simulink model "TX_PM_MODEL"  (R2024a)
settings: Solver=VariableStepAuto  StartTime=0.0  StopTime=1e-3  FixedStep=1e-9  RelTol=1e-3
values from neighbouring files (symbols this model uses):
  Cs = 12.5e-12    (= 1.25e-11)    [Oscillator_Setup.m]
  deltaVOSC = 0.5    [Oscillator_Setup.m]
  I0 = 100e-6    (= 0.0001)    [Oscillator_Setup.m]
  R = 0.2    [TX_PM_MODEL_Setup.m]
  Rf = 1e9    (= 1000000000)    [Oscillator_Setup.m]
  VDD = 5    [Oscillator_Setup.m]    (also in TX_PM_MODEL_Setup.m = 10)
  Vh = VDD - deltaVOSC    (= 4.5)    [Oscillator_Setup.m]
  Vl = deltaVOSC    (= 0.5)    [Oscillator_Setup.m]
undefined symbols (not defined in the file or in its folder): VDD_DRIVE
libraries: fl_lib x12, nesl_utility x7, ee_lib x1, dspsigops x1, spsTriangleGeneratorLib x1
settings Model: Creator=cian.odonnell  LastModifiedBy=cian.odonnell
settings SolverCC: EnableFixedStepZeroCrossing=on

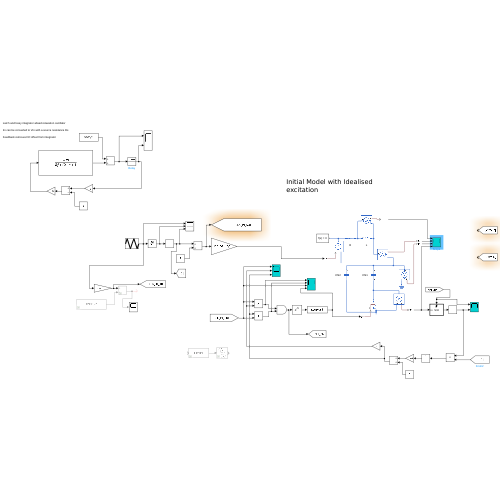
[thumbnail: Simulink's stored preview of the top-level diagram]
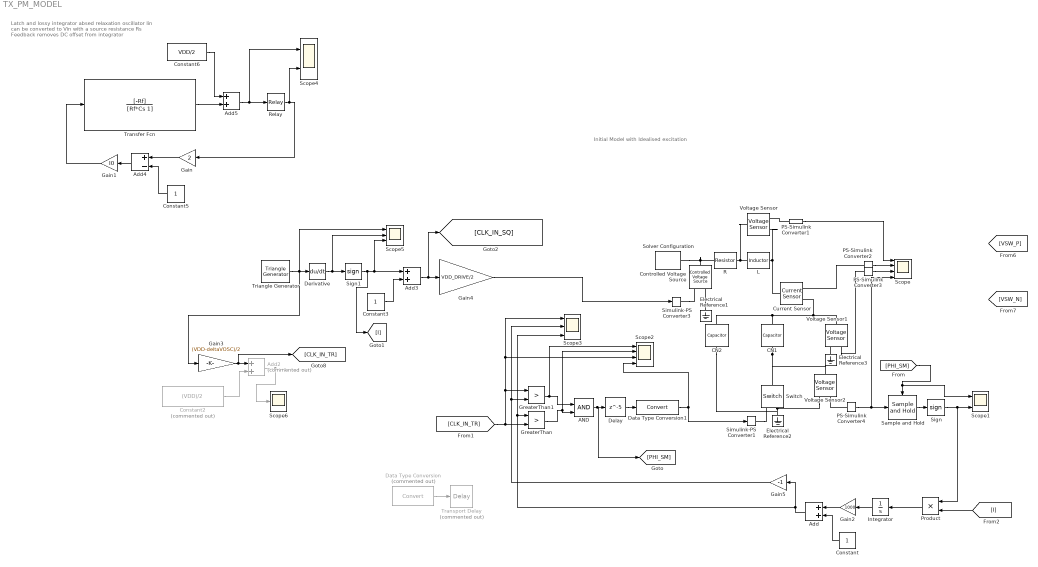
== system TX_PM_MODEL ==
  note: Initial Model with Idealised excitation
  note: Latch and lossy integrator absed relaxation oscillator
      |
      | Iin can be converted to Vin with a source resistance Rs
      |
      | Feedback removes DC offset from integrator
  AND : Logic  IconShape=distinctive  AllPortsSameDT=off  OutDataTypeStr=boolean
  Add : Sum
  Add2 : Sum  Commented=on
  Add3 : Sum
  Add4 : Sum  Inputs=+-
  Add5 : Sum
  CN1 : fl_lib/Electrical/Electrical Elements/Capacitor  c=3e-9 F  r=1e-6 Ohm  g=0 1/Ohm  i_specify=off  i_priority=None  i=0 A  i_nominal_specify=off  i_nominal_value=1  i_nominal_unit=A  v_specify=off  v_priority=None  v=0 V  v_nominal_specify=off  v_nominal_value=1  v_nominal_unit=V  vc_specify=off  vc_priority=High  vc=0 V  vc_nominal_specify=off  vc_nominal_value=1  vc_nominal_unit=V
  CN2 : fl_lib/Electrical/Electrical Elements/Capacitor  c=3e-9 F  r=1e-6 Ohm  g=0 1/Ohm  i_specify=off  i_priority=None  i=0 A  i_nominal_specify=off  i_nominal_value=1  i_nominal_unit=A  v_specify=off  v_priority=None  v=0 V  v_nominal_specify=off  v_nominal_value=1  v_nominal_unit=V  vc_specify=off  vc_priority=High  vc=0 V  vc_nominal_specify=off  vc_nominal_value=1  vc_nominal_unit=V
  Constant : Constant
  Constant2 : Constant  Commented=on  Value=(VDD)/2
  Constant3 : Constant
  Constant5 : Constant
  Constant6 : Constant  Value=VDD/2
  Controlled Voltage Source : fl_lib/Electrical/Electrical Sources/Controlled Voltage Source
  Current Sensor : fl_lib/Electrical/Electrical Sensors/Current Sensor
  Data Type Conversion : DataTypeConversion  Commented=on  SaturateOnIntegerOverflow=off  RndMeth=Floor
  Data Type Conversion1 : DataTypeConversion  SaturateOnIntegerOverflow=off  RndMeth=Floor
  Delay : Delay  DelayLength=5  SampleTime=1e-9
  Derivative : Derivative
  Electrical Reference1 : fl_lib/Electrical/Electrical Elements/Electrical Reference
  Electrical Reference2 : fl_lib/Electrical/Electrical Elements/Electrical Reference
  Electrical Reference3 : fl_lib/Electrical/Electrical Elements/Electrical Reference
  Gain : Gain  Gain=2
  Gain1 : Gain  Gain=I0
  Gain2 : Gain  Gain=1000
  Gain3 : Gain  Gain=(VDD-deltaVOSC)/2
  Gain4 : Gain  Gain=VDD_DRIVE/2
  Gain5 : Gain  Gain=-1
  GreaterThan : RelationalOperator  Operator=>  OutDataTypeStr=boolean  RndMeth=Simplest  InputSameDT=off
  GreaterThan1 : RelationalOperator  Operator=>  OutDataTypeStr=boolean  RndMeth=Simplest  InputSameDT=off
  Integrator : Integrator
  L : ee_lib/Passive/Inductor  l=L H  enable_L_tol=ee.enum.toleranceApplication.none  L_tol=20  tol_distribution=ee.enum.toleranceDistribution.uniform  nSigma=4  r=0 Ohm  g=1e-9 1/Ohm  enable_operating_limits=ee.enum.enable.no  operating_limit_action=ee.enum.passive.reportOpLim.warn  max_working_current=1 A  power_rating=1 W  enable_faults=ee.enum.enable.no  fault_action=simscape.enum.assert.action.none  lambdaPercent=50  k_faulted=0.9999  turnsShort=ee.enum.passive.inductor.turnsShortOption.no  openCct=ee.enum.enable.no  groundShort=ee.enum.passive.inductor.groundShortOption.no  groundShortG=0 1/Ohm  tau_fault=1e-3 s  fault_trigger=ee.enum.faults.faultTrigger.temporal  t_fault=1 s  max_permissible_voltage=100 V  n_fail_on_voltage=1  max_permissible_current=1 A  t_fail_on_current=1 s  i_L_specify=off  i_L_priority=High  i_L=0 A  i_L_nominal_specify=off  i_L_nominal_value=1  i_L_nominal_unit=A  faulted_specify=off  faulted_priority=None  faulted=0
  PS-Simulink Converter{1..4} (4 alike) : nesl_utility/PS-Simulink Converter  PhysicalDomain=network_engine_domain  SubClassName=ps_output  LeftPortType=input  RightPortType=output  PseudoPeriodic=off  Frequencies=[]  VectorFormat=inherit  Unit=inherit  AffineConversion=off
  Product : Product
  R : fl_lib/Electrical/Electrical Elements/Resistor  R=R Ohm  i_specify=off  i_priority=None  i=0 A  i_nominal_specify=off  i_nominal_value=1  i_nominal_unit=A  v_specify=off  v_priority=None  v=0 V  v_nominal_specify=off  v_nominal_value=1  v_nominal_unit=V
  Relay : Relay  OnSwitchValue=Vh  OffSwitchValue=Vl
  Sample and Hold : dspsigops/Sample and Hold  trig=Rising edge  initCond=0  latchinput=off
  Scope : Scope  NumInputPorts=4
  Scope1 : Scope  NumInputPorts=2
  Scope2 : Scope  NumInputPorts=4
  Scope3 : Scope  NumInputPorts=3
  Scope4 : Scope  NumInputPorts=2
  Scope5 : Scope  NumInputPorts=3
  Scope6 : Scope
  Sign : Signum
  Sign1 : Signum
  Simulink-PS Converter1 : nesl_utility/Simulink-PS Converter  PhysicalDomain=network_engine_domain  SubClassName=ps_input  LeftPortType=input  RightPortType=output  PseudoPeriodic=off  Frequencies=[]  NoiseDistribution=none  NoiseParameters=[]  Unit=1  AffineConversion=off  FilteringAndDerivatives=provide  SimscapeFilterOrder=1  InputFilterTimeConstant=0.001  UdotUserProvided=0
  Simulink-PS Converter3 : nesl_utility/Simulink-PS Converter  PhysicalDomain=network_engine_domain  SubClassName=ps_input  LeftPortType=input  RightPortType=output  PseudoPeriodic=off  Frequencies=[]  NoiseDistribution=none  NoiseParameters=[]  Unit=1  AffineConversion=off  FilteringAndDerivatives=provide  SimscapeFilterOrder=1  InputFilterTimeConstant=0.001  UdotUserProvided=0
  Solver Configuration : nesl_utility/Solver Configuration  PhysicalDomain=network_engine_domain  SubClassName=solver  LeftPortType=input  RightPortType=generic  Tones=[]  Harmonics=[]  SimulateNoise=off  Profile=off  UseLocalSampling=off  EnableSwitchedLinearOptims=on  FrequencyDomain=off  UseCCode=off  RelTol=0.001  AbsTol=0.001  MinStep=1e-09  ToWorkspace=off  RevertToSquareIcSolve=off  NumHomotopyIterations=100  PhasorMode=off  PhasorModeNumHarmonics=1  ConsistencySolver=NEWTON_XTOL_AFTER_FTOL  IndexReductionMethod=DerivativeReplacement  DoDC=off  ResidualTolerance=1e-09  ConsistencyTolSource=GLOBAL  ConsistencyAbsTol=0.001  ConsistencyRelTol=0.001  ConsistencyTolFactor=0.001  UseLocalSolver=off  LocalSolverChoice=NE_BACKWARD_EULER_ADVANCER  ResolveIndetEquations=on  FunctionEvalNumThread=1  LocalSolverSampleTime=0.001  DoFixedCost=off  MaxNonlinIter=3  MaxModeIter=2  ComputeImpulses=off  ImpulseIterations=2  LinearAlgebra=auto  LinearAlgebraNumThread=0  EquationFormulation=NE_TIME_EF  DelaysMemoryBudget=1024  AutomaticFiltering=on  FilteringTimeConstant=0.001  PartitionStorageMethod=AS_NEEDED  PartitionMemoryBudget=1024  PartitionMethod=ROBUST  MultibodyUseLocalSolver=off  MultibodyLocalSolverChoice=ODE1  MultibodyLocalSolverSampleTime=0.001
  Switch : fl_lib/Electrical/Electrical Elements/Switch  R_closed=0.01 Ohm  G_open=1e-8 1/Ohm  Threshold=0.5  i_specify=off  i_priority=None  i=0 A  i_nominal_specify=off  i_nominal_value=1  i_nominal_unit=A  v_specify=off  v_priority=None  v=0 V  v_nominal_specify=off  v_nominal_value=1  v_nominal_unit=V
  Transfer Fcn : TransferFcn  Numerator=[-Rf]  Denominator=[Rf*Cs 1]
  Transport Delay : TransportDelay  Commented=on  DelayTime=1e-9
  Triangle Generator : spsTriangleGeneratorLib/Triangle Generator  Freq=fin  Phase=90  Ts=0
  Voltage Sensor : fl_lib/Electrical/Electrical Sensors/Voltage Sensor
  Voltage Sensor1 : fl_lib/Electrical/Electrical Sensors/Voltage Sensor
  Voltage Sensor2 : fl_lib/Electrical/Electrical Sensors/Voltage Sensor
  wires:
  PS-Simulink Converter2/1 -> Scope/2
  PS-Simulink Converter1/1 -> Scope/1
  PS-Simulink Converter3/1 -> Scope/3
  GreaterThan/1 -> Scope2/2, AND/2
  PS-Simulink Converter4/1 -> Sample and Hold/1, Scope/4
  Sample and Hold/1 -> Sign/1
  [PHI_SM] -> Scope1/1, Sample and Hold/Trigger
  Add5/1 -> Scope4/1, Relay/1
  Transfer Fcn/1 -> Add5/2
  Gain1/1 -> Transfer Fcn/1
  Add4/1 -> Gain1/1
  Gain/1 -> Add4/1
  Constant5/1 -> Add4/2
  Constant6/1 -> Add5/1
  Relay/1 -> Gain/1, Scope4/2
  Add2/1 -> Scope6/1
  Gain3/1 -> [CLK_IN_TR], Add2/1
  Triangle Generator/1 -> Gain3/1, Scope5/1, Derivative/1
  Derivative/1 -> Sign1/1, Scope5/2
  Sign1/1 -> [I], Add3/1, Scope5/3
  Constant2/1 -> Add2/2
  Constant3/1 -> Add3/2
  Add3/1 -> [CLK_IN_SQ], Gain4/1
  Gain4/1 -> Simulink-PS Converter3/1
  [CLK_IN_TR] -> GreaterThan/2, GreaterThan1/1, Scope3/1, Scope2/3
  Integrator/1 -> Gain2/1
  Data Type Conversion/1 -> Transport Delay/1
  Gain5/1 -> GreaterThan1/2, Scope3/2
  GreaterThan1/1 -> Scope2/1, AND/1
  Data Type Conversion1/1 -> Simulink-PS Converter1/1, Scope2/4
  AND/1 -> [PHI_SM], Delay/1
  Delay/1 -> Data Type Conversion1/1
  Sign/1 -> Product/1, Scope1/2
  Product/1 -> Integrator/1
  Add/1 -> GreaterThan/1, Scope3/3, Gain5/1
  [I] -> Product/2
  Gain2/1 -> Add/1
  Constant/1 -> Add/2
  connections:
  Controlled Voltage Source/LConn1 -- R/LConn1 -- Solver Configuration/RConn1
  Simulink-PS Converter3/RConn1 -- Controlled Voltage Source/RConn1
  Electrical Reference1/LConn1 -- Controlled Voltage Source/RConn2
  Current Sensor/LConn1 -- Voltage Sensor/RConn2 -- L/RConn1
  CN1/LConn1 -- Voltage Sensor1/LConn1 -- Current Sensor/RConn2 -- CN2/LConn1
  PS-Simulink Converter2/LConn1 -- Current Sensor/RConn1
  CN1/RConn1 -- Voltage Sensor2/LConn1 -- Switch/LConn1
  L/LConn1 -- Voltage Sensor/LConn1 -- R/RConn1
  PS-Simulink Converter1/LConn1 -- Voltage Sensor/RConn1
  Voltage Sensor1/RConn1 -- PS-Simulink Converter3/LConn1
  Electrical Reference2/LConn1 -- CN2/RConn1 -- Switch/RConn2 -- Voltage Sensor2/RConn2
  Simulink-PS Converter1/RConn1 -- Switch/RConn1
  PS-Simulink Converter4/LConn1 -- Voltage Sensor2/RConn1
  Electrical Reference3/LConn1 -- Voltage Sensor1/RConn2
